simulink model "ssc_mass_spring_damper_sl"  (R2021a)
settings: Solver=VariableStepAuto  StartTime=0.0  StopTime=5  MaxStep=0.025  RelTol=1e-3  AbsTol=1e-3  EnableMultiTasking=on
PreLoadFcn:
  | m = 3.600;     % kg
  | k = 400;    % N/m
  | b = 10;      % Ns/m
  | x0=1; %m
values from neighbouring files (symbols this model uses):
  F = ones(size(t1))    [hw2p5.m]    (also in massSpringDamper.m = 1)
libraries: fl_lib x6, nesl_utility x2
CloseFcn:
  | try,close(h1_ssc_mass_spring_damper_sl),end
  | clear h1_ssc_mass_spring_damper_sl
  | 
  | clear simlog_ssc_mass_spring_damper_sl
  | clear logsout_ssc_mass_spring_damper_sl
Description:
  | Mass-Spring-Damper in Simulink(R) and Simscape(TM)
settings Model: Creator=The MathWorks, Inc.  LastModifiedBy=Zeke
settings SolverCC: AutoScaleAbsTol=off  AlgebraicLoopSolver=TrustRegion
settings DataIOCC: LimitDataPoints=on  SaveFormat=Array  ReturnWorkspaceOutputs=off  SignalLoggingName=logsout_ssc_mass_spring_damper_sl
settings OptimizationCC: LifeSpan=inf
settings DebuggingCC: SolverPrmCheckMsg=warning  AllowSymbolicDim=off  PregeneratedLibrarySubsystemCodeDiagnostic=none  SFUnexpectedBacktrackingDiag=warning  SFNoUnconditionalDefaultTransitionDiag=warning  SFExecutionAtInitializationDiag=none  SFMachineParentedDataDiag=warning  ArithmeticOperatorsInVariantConditions=warning
settings HardwareCC: ProdBitPerPointer=32  ProdBitPerSizeT=32  ProdBitPerPtrDiffT=32  ProdLargestAtomicFloat=None  ProdIntDivRoundTo=Undefined  ProdEndianess=Unspecified  ProdWordSize=32  ProdHWDeviceType=32-bit Generic
settings ModelReferenceCC: PropagateSignalLabelsOutOfModel=off
settings SFSimCC: SimUseLocalCustomCode=off  CustomCodeUndefinedFunction=UseInterfaceOnly
settings RTWCC: RTWUseLocalCustomCode=off
settings CodeAppCC: StateflowObjectComments=on
settings GRTTargetCC: TargetLangStandard=C89/C90 (ANSI)
settings ConfigComp: CovMetricSettings=dw  CovSaveCumulativeToWorkspaceVar=on  CovSaveSingleToWorkspaceVar=on  CovExternalEMLEnable=off  CovSFcnEnable=off
settings SimscapeCC: SimscapeLogType=all  SimscapeLogSimulationStatistics=on  SimscapeLogName=simlog_ssc_mass_spring_damper_sl  SimscapeLogDataHistory=10000

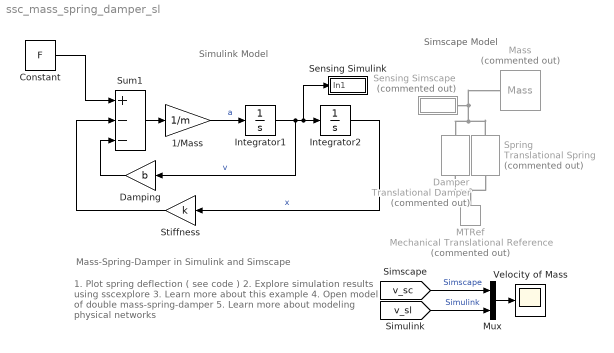
== system ssc_mass_spring_damper_sl ==
  note: 1. Plot spring deflection ( see code )
      | 2. Explore simulation results using sscexplore
      | 3. Learn more about this example
      | 4. Open model of double mass-spring-damper
      | 5. Learn more about modeling physical networks
  note: Mass-Spring-Damper in Simulink and Simscape
  note: Simulink Model
  note: Simscape Model
  "1/Mass " : Gain  Gain=1/m  SaturateOnIntegerOverflow=on  OutDataTypeStr=Inherit: Same as input  ParamDataTypeStr=Inherit: Same as input
  Constant : Constant  Value=F
  Damper : fl_lib/Mechanical/Translational Elements/Translational Damper  Commented=on  D=b N/(m/s)  v_specify=off  v_priority=High  v=0 m/s  v_nominal_specify=off  v_nominal_unit=m/s  v_nominal_value=1  f_specify=off  f_priority=High  f=0 N  f_nominal_specify=off  f_nominal_unit=N  f_nominal_value=1
  Damping : Gain  Gain=b  SaturateOnIntegerOverflow=on  OutDataTypeStr=Inherit: Same as input  ParamDataTypeStr=Inherit: Same as input
  Integrator1 : Integrator
  Integrator2 : Integrator  InitialCondition=1
      settings: AttributesFormatString=x0 = %<InitialCondition> m
  MTRef : fl_lib/Mechanical/Translational Elements/Mechanical Translational Reference  Commented=on
  Mass : fl_lib/Mechanical/Translational Elements/Mass  Commented=on  mass=m kg  num_ports=foundation.enum.numPorts2.one  v_specify=off  v_priority=High  v=0 m/s  v_nominal_specify=off  v_nominal_unit=m/s  v_nominal_value=1  f_specify=off  f_priority=High  f=0 N  f_nominal_specify=off  f_nominal_unit=N  f_nominal_value=1
  Mux : Mux  Inputs=2
  Sensing Simscape : Subsystem  Commented=on
      mask Display: disp('v_sc')
  Sensing Simulink : Subsystem
      mask Display: disp('v_sl')
  Spring : fl_lib/Mechanical/Translational Elements/Translational Spring  Commented=on  spr_rate=k N/m  v_specify=off  v_priority=High  v=0 m/s  v_nominal_specify=off  v_nominal_unit=m/s  v_nominal_value=1  f_specify=off  f_priority=High  f=0 N  f_nominal_specify=off  f_nominal_unit=N  f_nominal_value=1  x_specify=on  x_priority=High  x=1 m  x_nominal_specify=off  x_nominal_unit=m  x_nominal_value=1
      settings: AttributesFormatString=x0 = %<x> %<x_unit>
  Stiffness : Gain  Gain=k  SaturateOnIntegerOverflow=on  OutDataTypeStr=Inherit: Same as input  ParamDataTypeStr=Inherit: Same as input
  Sum1 : Sum  Inputs=+--  InputSameDT=on  SaturateOnIntegerOverflow=on  OutDataTypeStr=Inherit: Same as first input
  Velocity of Mass : Scope
  wires:
  "1/Mass "/1 -> Integrator1/1  "a"
  Sum1/1 -> "1/Mass "/1
  Damping/1 -> Sum1/3
  Stiffness/1 -> Sum1/2
  Integrator2/1 -> Stiffness/1  "x"
  Integrator1/1 -> Sensing Simulink/1(In1), Integrator2/1, Damping/1  "v"
  Mux/1 -> Velocity of Mass/1
  [v_sc] -> Mux/1  "Simscape"
  [v_sl] -> Mux/2  "Simulink"
  Constant/1 -> Sum1/1
  connections:
  Spring/RConn1 -- Damper/RConn1 -- MTRef/LConn1
  Spring/LConn1 -- Sensing Simscape/LConn1 -- Mass/LConn1 -- Damper/LConn1

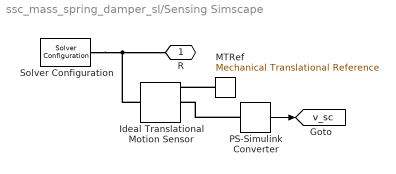
== system ssc_mass_spring_damper_sl/Sensing Simscape ==
  Ideal Translational Motion Sensor : fl_lib/Mechanical/Mechanical Sensors/Ideal Translational Motion Sensor  offset=1 m
  MTRef : fl_lib/Mechanical/Translational Elements/Mechanical Translational Reference
  PS-Simulink Converter : nesl_utility/PS-Simulink Converter  PhysicalDomain=network_engine_domain  SubClassName=ps_output  LeftPortType=input  RightPortType=output  PseudoPeriodic=off  Frequencies=[]  Unit=1  AffineConversion=off
      settings: SourceProductBaseCode=PW,SS
  Solver Configuration : nesl_utility/Solver Configuration  PhysicalDomain=network_engine_domain  SubClassName=solver  LeftPortType=input  RightPortType=generic  Tones=[]  Harmonics=[]  SimulateNoise=off  Profile=off  UseLocalSampling=off  EnableSwitchedLinearOptims=on  FrequencyDomain=off  UseCCode=off  RelTol=0.001  AbsTol=1e-06  MinStep=1e-09  ToWorkspace=off  RevertToSquareIcSolve=off  NumHomotopyIterations=100  PhasorMode=off  PhasorModeNumHarmonics=1  DoDC=off  ResidualTolerance=1e-9  UseLocalSolver=off  LocalSolverChoice=NE_BACKWARD_EULER_ADVANCER  LocalSolverSampleTime=.001  DoFixedCost=off  MaxNonlinIter=12  MaxModeIter=2  ComputeImpulses=off  ImpulseIterations=2  LinearAlgebra=auto  EquationFormulation=NE_TIME_EF  DelaysMemoryBudget=1024  AutomaticFiltering=on  FilteringTimeConstant=0.001  PartitionStorageMethod=AS_NEEDED  PartitionMemoryBudget=1024  PartitionMethod=FAST
      settings: SourceProductBaseCode=PW,SS
  R : PMIOPort  Side=Left
  tag scope: v_sc=global
  wires:
  PS-Simulink Converter/1 -> [v_sc]
  connections:
  Solver Configuration/RConn1 -- Ideal Translational Motion Sensor/LConn1 -- R/RConn1
  PS-Simulink Converter/LConn1 -- Ideal Translational Motion Sensor/RConn2
  MTRef/LConn1 -- Ideal Translational Motion Sensor/RConn1

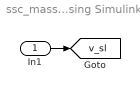
== system ssc_mass_spring_damper_sl/Sensing Simulink ==
  In1 : Inport
  tag scope: v_sl=global
  wires:
  In1/1 -> [v_sl]
